simulink subsystem "Phase"  (R2021b)
settings: Solver=VariableStepAuto  StartTime=0.0  StopTime=10.0  RelTol=1e-3
libraries: matrix_library x1
settings Model: Creator=austm  LastModifiedBy=austm

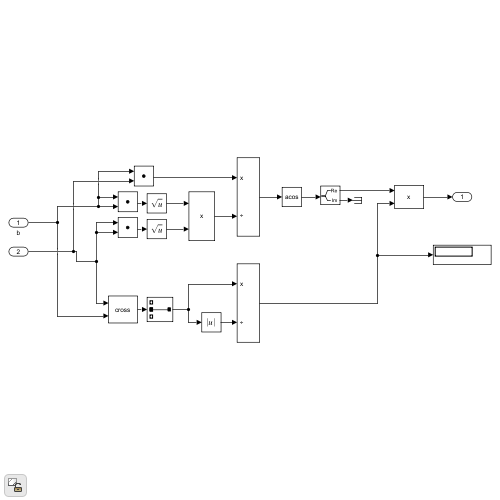
[thumbnail: Simulink's stored preview of the top-level diagram]
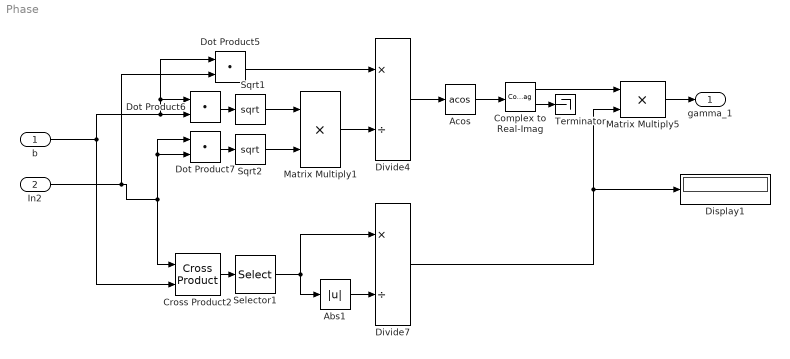
== system Phase ==
  b : Inport
  In2 : Inport  Port=2
  Abs1 : Abs
  Acos : Trigonometry  Operator=acos  OutputSignalType=complex
  Complex to Real-Imag : ComplexToRealImag
  Cross Product2 : matrix_library/Cross Product
      settings: SourceProductBaseCode=SL
  Display1 : Display
  Divide4 : Product  Inputs=*/
  Divide7 : Product  Inputs=*/
  Dot Product5 : DotProduct  InputSameDT=on  OutDataTypeStr=Inherit: Inherit via internal rule
  Dot Product6 : DotProduct  InputSameDT=on  OutDataTypeStr=Inherit: Inherit via internal rule
  Dot Product7 : DotProduct  InputSameDT=on  OutDataTypeStr=Inherit: Inherit via internal rule
  Matrix Multiply1 : Product
  Matrix Multiply5 : Product
  Selector1 : Selector  InputPortWidth=3  IndexOptions=Index vector (dialog)  Indices=1  OutputSizes=1
  Sqrt1 : Sqrt  SaturateOnIntegerOverflow=on
  Sqrt2 : Sqrt  SaturateOnIntegerOverflow=on
  Terminator : Terminator
  gamma_1 : Outport
  wires:
  Matrix Multiply5/1 -> gamma_1/1
  Sqrt1/1 -> Matrix Multiply1/1
  Dot Product5/1 -> Divide4/1
  b/1 -> Dot Product6/2, Dot Product6/1, Dot Product5/1, Cross Product2/2
  In2/1 -> Dot Product7/2, Dot Product7/1, Cross Product2/1, Dot Product5/2
  Matrix Multiply1/1 -> Divide4/2
  Selector1/1 -> Abs1/1, Divide7/1
  Sqrt2/1 -> Matrix Multiply1/2
  Complex to Real-Imag/1 -> Matrix Multiply5/1
  Dot Product7/1 -> Sqrt2/1
  Dot Product6/1 -> Sqrt1/1
  Cross Product2/1 -> Selector1/1
  Abs1/1 -> Divide7/2
  Divide4/1 -> Acos/1
  Acos/1 -> Complex to Real-Imag/1
  Complex to Real-Imag/2 -> Terminator/1
  Divide7/1 -> Matrix Multiply5/2, Display1/1
